simulink library "Valve_ThermoTset"  (Simulink 8.2)
settings: Solver=ode45  StartTime=0.0  StopTime=10.0  RelTol=1e-3
libraries: carnot x1
settings Model: Creator=lena.frank  LastModifiedBy=drhf

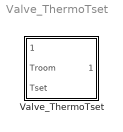
== system Valve_ThermoTset ==
  Valve_ThermoTset : Subsystem  mask(thermostatic valve){p=3, op=0.5, bl=10, ts=30, dia=0.02, vpos=[0 0.1 1], vqua=[1e6 1e6 1]}
      mask prompts: p "proportional Range [K]"; op "operating point [0..1] (valve position at set temperature)"; bl "play hysteresis []"; ts "first-order hold ts [s]"; dia "diameter [m]"; vpos "Valve position vector [0..1]"; vqua "Vector with quadratic pressure drop in massflow in Pa*s²/kg²"
      mask help:
      | Thermostatic valve for a radiator.
      | set temperature and slope
      | valve position = -slope * (T(sensor) - Toffset)
      mask init:
      | % p=1/p;
      | % op = min(1, max(0, op));
      | % tu = max(tu,0);
      | % ts = max(ts,0);
      | % dia = max(dia, 0.001);
      | %
      mask Help: web(fullfile(path_carnot('help'),'Valve_Thermostatic.html'),'-helpbrowser')
      mask Display:
      | plot(-30,-10,130,110,[20,80,80,20,20],[60,30,60,30,60],[50,50],[45,70],[60,40],[96,96],[50,50],[75,96])
      | port_label('input',1,'THB')
      | port_label('input',2,'Troom')
      | port_label('input',3,'Tset')
      | port_label('output',1,'THB')

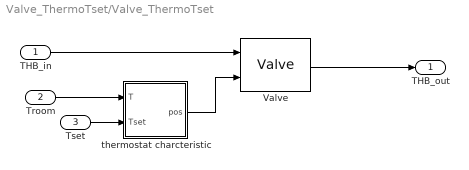
== system Valve_ThermoTset/Valve_ThermoTset ==
  THB_in : Inport
  Troom : Inport  Port=2
  Tset : Inport  Port=3
  Valve : carnot/Hydraulics/Valve  pos_values=vpos  dp_values=vqua
  thermostat charcteristic : Subsystem
  THB_out : Outport
  wires:
  thermostat charcteristic/1(pos) -> Valve/2
  Valve/1 -> THB_out/1
  THB_in/1 -> Valve/1
  Tset/1 -> thermostat charcteristic/2(Tset)
  Troom/1 -> thermostat charcteristic/1(T)

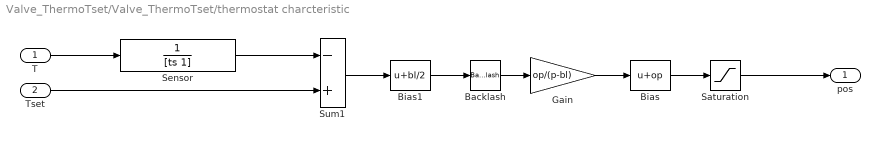
== system Valve_ThermoTset/Valve_ThermoTset/thermostat charcteristic ==
  T : Inport
  Tset : Inport  Port=2
  Backlash : Backlash  BacklashWidth=bl
  Bias : Bias  Bias=op
  Bias1 : Bias  Bias=bl/2
  Gain : Gain  Gain=op/(p-bl)
  Saturation : Saturate  UpperLimit=1  LowerLimit=0
  Sensor : TransferFcn  Denominator=[ts 1]
  Sum1 : Sum  Inputs=-+  SaturateOnIntegerOverflow=on  InputSameDT=on  OutDataTypeStr=Inherit: Same as first input
  pos : Outport  InitialOutput=0
  wires:
  Sensor/1 -> Sum1/1
  Bias1/1 -> Backlash/1
  Gain/1 -> Bias/1
  Backlash/1 -> Gain/1
  Sum1/1 -> Bias1/1
  Saturation/1 -> pos/1
  Bias/1 -> Saturation/1
  T/1 -> Sensor/1
  Tset/1 -> Sum1/2
